simulink model "B_14"  (R2018b)
settings: Solver=VariableStepAuto  StartTime=0.0  StopTime=1  MaxStep=1e-4  RelTol=1e-6
StopFcn:
  | %CELEC_plot;
settings Model: Creator=Administrator  LastModifiedBy=Administrator

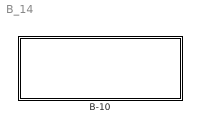
== system B_14 ==
  B-10 : Subsystem  mask{Vset=10, R=2, L=0.02, J=10, KE=1.8, KT=17.2}
      mask prompts: Vset "电源电压(V)"; R "电枢电阻(Ω）"; L "电枢电感(H)"; J "转动惯量(kg.m^3)"; KE "反电势系数(V/rpm)"; KT "电磁转矩系数(N.m/A)"

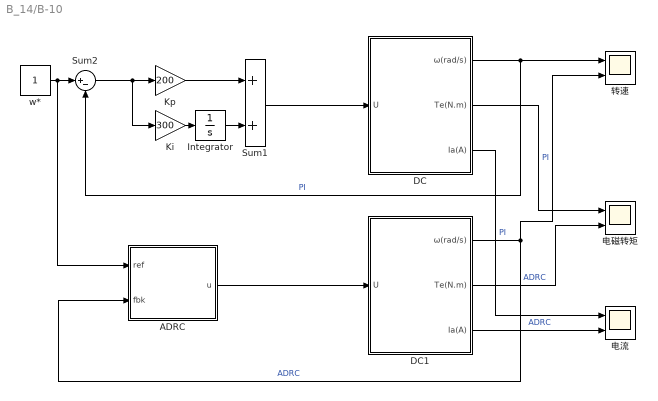
== system B_14/B-10 ==
  ADRC : Subsystem  mask{alpha0=0.95, delta0=0.01, r0=9000, alpha1=0.95, delta1=0.01, beta1=10000, beta2=100000, alpha2=0.95, delta2=0.01, b0=100, k=1000}
      mask prompts: alpha0 "跟踪因子α"; delta0 "滤波因子δ"; r0 "速度因子r0"; alpha1 "跟踪因子α"; delta1 "滤波因子δ"; beta1 "校正增益β1"; beta2 "校正增益β2"; alpha2 "跟踪因子α"; delta2 "滤波因子δ"; b0 "补偿因子b0"; k "调节增益k"
      mask DialogControl Container3 Prompt: TD
      mask DialogControl Container4 Prompt: ESO
      mask DialogControl Container5 Prompt: NLSEF
  DC : Subsystem
  DC1 : Subsystem
  Integrator : Integrator
  Ki : Gain  Gain=300
  Kp : Gain  Gain=200
  Sum1 : Sum
  Sum2 : Sum  Inputs=|+-
  w* : Constant
  电流 : Scope  NumInputPorts=2
  电磁转矩 : Scope  NumInputPorts=2
  转速 : Scope  NumInputPorts=2
  wires:
  Sum2/1 -> Ki/1, Kp/1
  Kp/1 -> Sum1/1
  Ki/1 -> Integrator/1
  Integrator/1 -> Sum1/2
  DC/1(ω(rad/s)) -> 转速/1, Sum2/2  "PI"
  Sum1/1 -> DC/1(U)
  DC/2(Te(N.m)) -> 电磁转矩/1  "PI"
  DC/3(Ia(A)) -> 电流/1  "PI"
  ADRC/1(u) -> DC1/1(U)
  DC1/2(Te(N.m)) -> 电磁转矩/2  "ADRC"
  DC1/1(ω(rad/s)) -> ADRC/2(fbk), 转速/2  "ADRC"
  DC1/3(Ia(A)) -> 电流/2  "ADRC"
  w*/1 -> ADRC/1(ref), Sum2/1

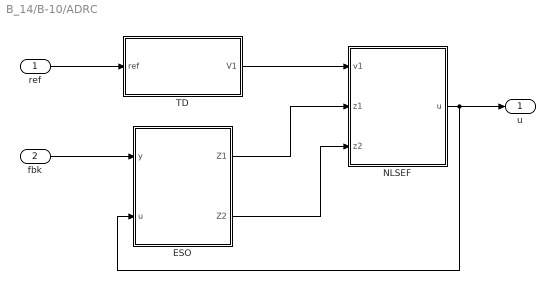
== system B_14/B-10/ADRC ==
  ref : Inport
  fbk : Inport  Port=2
  ESO : Subsystem
  NLSEF : Subsystem
  TD : Subsystem
  u : Outport
  wires:
  NLSEF/1(u) -> u/1, ESO/2(u)
  ESO/1("Z1   ") -> NLSEF/2(z1)
  ref/1 -> TD/1(ref)
  ESO/2(Z2) -> NLSEF/3(z2)
  TD/1(V1) -> NLSEF/1(v1)
  fbk/1 -> ESO/1(y)

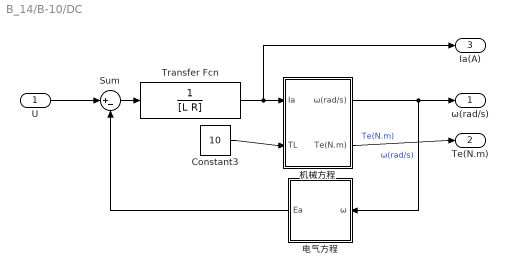
== system B_14/B-10/DC ==
  U : Inport
  Constant3 : Constant  Value=10
  Sum : Sum  Inputs=|+-
  Transfer Fcn : TransferFcn  Denominator=[L R]
  机械方程 : Subsystem
  电气方程 : Subsystem
  ω(rad/s) : Outport
  Te(N.m) : Outport  Port=2
  Ia(A) : Outport  Port=3
  wires:
  Transfer Fcn/1 -> Ia(A)/1, 机械方程/1(Ia)
  Constant3/1 -> 机械方程/2(TL)
  Sum/1 -> Transfer Fcn/1
  机械方程/1(ω(rad/s)) -> 电气方程/1(ω), ω(rad/s)/1  "ω(rad/s)"
  电气方程/1(Ea) -> Sum/2
  U/1 -> Sum/1
  机械方程/2(Te(N.m)) -> Te(N.m)/1  "Te(N.m)"

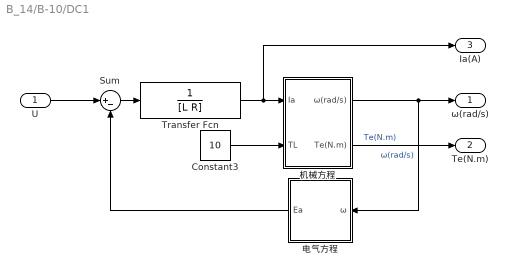
== system B_14/B-10/DC1 ==
  U : Inport
  Constant3 : Constant  Value=10
  Sum : Sum  Inputs=|+-
  Transfer Fcn : TransferFcn  Denominator=[L R]
  机械方程 : Subsystem
  电气方程 : Subsystem
  ω(rad/s) : Outport
  Te(N.m) : Outport  Port=2
  Ia(A) : Outport  Port=3
  wires:
  Transfer Fcn/1 -> Ia(A)/1, 机械方程/1(Ia)
  Constant3/1 -> 机械方程/2(TL)
  Sum/1 -> Transfer Fcn/1
  机械方程/1(ω(rad/s)) -> 电气方程/1(ω), ω(rad/s)/1  "ω(rad/s)"
  电气方程/1(Ea) -> Sum/2
  U/1 -> Sum/1
  机械方程/2(Te(N.m)) -> Te(N.m)/1  "Te(N.m)"

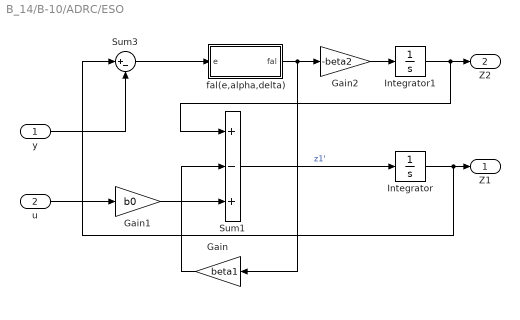
== system B_14/B-10/ADRC/ESO ==
  y : Inport
  u : Inport  Port=2
  Gain : Gain  Gain=beta1
  Gain1 : Gain  Gain=b0
  Gain2 : Gain  Gain=-beta2
  Integrator : Integrator
  Integrator1 : Integrator
  Sum1 : Sum  Inputs=+-+
  Sum3 : Sum  Inputs=|+-
  fal(e,alpha,delta) : Subsystem  mask{alpha=alpha1, delta=delta1}
      mask prompts: alpha "跟踪因子α"; delta "滤波因子δ"
  "Z1   " : Outport
  Z2 : Outport  Port=2
  wires:
  fal(e,alpha,delta)/1(fal) -> Gain2/1, Gain/1
  Sum3/1 -> fal(e,alpha,delta)/1(e)
  y/1 -> Sum3/2
  Integrator/1 -> Sum3/1, "Z1   "/1
  Sum1/1 -> Integrator/1  "z1'"
  Gain/1 -> Sum1/2
  u/1 -> Gain1/1
  Gain1/1 -> Sum1/3
  Gain2/1 -> Integrator1/1
  Integrator1/1 -> Z2/1, Sum1/1

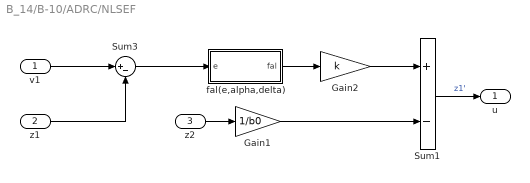
== system B_14/B-10/ADRC/NLSEF ==
  v1 : Inport
  z1 : Inport  Port=2
  z2 : Inport  Port=3
  Gain1 : Gain  Gain=1/b0
  Gain2 : Gain  Gain=k
  Sum1 : Sum  Inputs=+-
  Sum3 : Sum  Inputs=|+-
  fal(e,alpha,delta) : Subsystem  mask{alpha=alpha2, delta=delta2}
      mask prompts: alpha "跟踪因子α"; delta "滤波因子δ"
  u : Outport
  wires:
  fal(e,alpha,delta)/1(fal) -> Gain2/1
  Sum3/1 -> fal(e,alpha,delta)/1(e)
  v1/1 -> Sum3/1
  Gain2/1 -> Sum1/1
  z1/1 -> Sum3/2
  Gain1/1 -> Sum1/2
  z2/1 -> Gain1/1
  Sum1/1 -> u/1  "z1'"

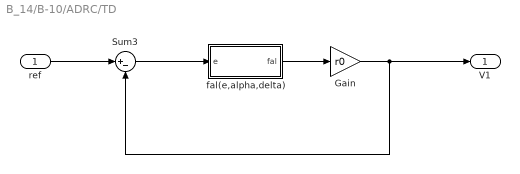
== system B_14/B-10/ADRC/TD ==
  ref : Inport
  Gain : Gain  Gain=r0
  Sum3 : Sum  Inputs=|+-
  fal(e,alpha,delta) : Subsystem  mask{alpha=alpha0, delta=delta0}
      mask prompts: alpha "跟踪因子α"; delta "滤波因子δ"
  V1 : Outport
  wires:
  fal(e,alpha,delta)/1(fal) -> Gain/1
  Sum3/1 -> fal(e,alpha,delta)/1(e)
  ref/1 -> Sum3/1
  Gain/1 -> V1/1, Sum3/2

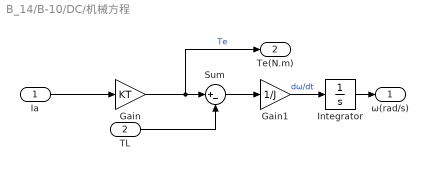
== system B_14/B-10/DC/机械方程 ==
  Ia : Inport
  TL : Inport  Port=2
  Gain : Gain  Gain=KT
  Gain1 : Gain  Gain=1/J
  Integrator : Integrator
  Sum : Sum  Inputs=|+-
  ω(rad/s) : Outport
  Te(N.m) : Outport  Port=2
  wires:
  Gain1/1 -> Integrator/1  "dω/dt"
  Sum/1 -> Gain1/1
  Gain/1 -> Te(N.m)/1, Sum/1  "Te"
  TL/1 -> Sum/2
  Ia/1 -> Gain/1
  Integrator/1 -> ω(rad/s)/1

== system B_14/B-10/DC/电气方程 ==
  ω : Inport
  V/rpm : Gain  Gain=KE
  rad/s 2 rpm : Gain  Gain=30/pi
  Ea : Outport
  wires:
  rad/s 2 rpm/1 -> V/rpm/1
  ω/1 -> rad/s 2 rpm/1
  V/rpm/1 -> Ea/1

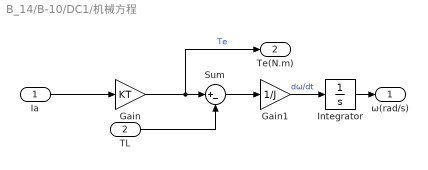
== system B_14/B-10/DC1/机械方程 ==
  Ia : Inport
  TL : Inport  Port=2
  Gain : Gain  Gain=KT
  Gain1 : Gain  Gain=1/J
  Integrator : Integrator
  Sum : Sum  Inputs=|+-
  ω(rad/s) : Outport
  Te(N.m) : Outport  Port=2
  wires:
  Gain1/1 -> Integrator/1  "dω/dt"
  Sum/1 -> Gain1/1
  Gain/1 -> Te(N.m)/1, Sum/1  "Te"
  TL/1 -> Sum/2
  Ia/1 -> Gain/1
  Integrator/1 -> ω(rad/s)/1

== system B_14/B-10/DC1/电气方程 ==
  ω : Inport
  V/rpm : Gain  Gain=KE
  rad/s 2 rpm : Gain  Gain=30/pi
  Ea : Outport
  wires:
  rad/s 2 rpm/1 -> V/rpm/1
  ω/1 -> rad/s 2 rpm/1
  V/rpm/1 -> Ea/1

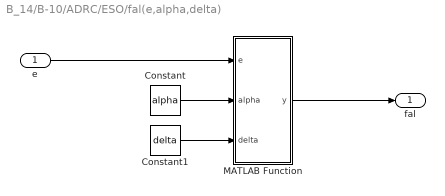
== system B_14/B-10/ADRC/ESO/fal(e,alpha,delta) ==
  e : Inport
  Constant : Constant  Value=alpha
  Constant1 : Constant  Value=delta
  MATLAB Function : MATLAB Function  TreatAsAtomicUnit=on
  fal : Outport
  wires:
  Constant1/1 -> MATLAB Function/3(delta)
  MATLAB Function/1(y) -> fal/1
  Constant/1 -> MATLAB Function/2(alpha)
  e/1 -> MATLAB Function/1(e)

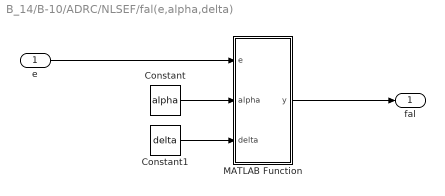
== system B_14/B-10/ADRC/NLSEF/fal(e,alpha,delta) ==
  e : Inport
  Constant : Constant  Value=alpha
  Constant1 : Constant  Value=delta
  MATLAB Function : MATLAB Function  TreatAsAtomicUnit=on
  fal : Outport
  wires:
  Constant1/1 -> MATLAB Function/3(delta)
  MATLAB Function/1(y) -> fal/1
  Constant/1 -> MATLAB Function/2(alpha)
  e/1 -> MATLAB Function/1(e)

== system B_14/B-10/ADRC/TD/fal(e,alpha,delta) ==
  e : Inport
  Constant : Constant  Value=alpha
  Constant1 : Constant  Value=delta
  MATLAB Function : MATLAB Function  TreatAsAtomicUnit=on
  fal : Outport
  wires:
  Constant1/1 -> MATLAB Function/3(delta)
  MATLAB Function/1(y) -> fal/1
  Constant/1 -> MATLAB Function/2(alpha)
  e/1 -> MATLAB Function/1(e)

== matlab function B_14/B-10/ADRC/ESO/fal(e,alpha,delta)/MATLAB Function ==
  data: e input; y output; alpha input; delta input
function y = fcn(e,alpha,delta)

if abs(e) > delta
    y = ( abs(e) )^ alpha*sign(e);
else
    y = e/(delta^(1-alpha));
end

end

== matlab function B_14/B-10/ADRC/TD/fal(e,alpha,delta)/MATLAB Function ==
  data: e input; y output; alpha input; delta input
function y = fcn(e,alpha,delta)

if abs(e) > delta
    y = ( abs(e) )^ alpha*sign(e);
else
    y = e/(delta^(1-alpha));
end

end

== matlab function B_14/B-10/ADRC/NLSEF/fal(e,alpha,delta)/MATLAB Function ==
  data: e input; y output; alpha input; delta input
function y = fcn(e,alpha,delta)

if abs(e) > delta
    y = ( abs(e) )^ alpha*sign(e);
else
    y = e/(delta^(1-alpha));
end

end
